simulink model "hp_v2"  (R2024b)
settings: Solver=VariableStepAuto  StartTime=0.0  StopTime=tf  MaxStep=1e-4  RelTol=1e-4  AbsTol=1e-4
values from neighbouring files (symbols this model uses):
  base = hexapod.base    [calcHomePose.m]    (also in calcMotorAngles.m; calcMotorAngles2.m; fk_z.m; ik_hexapod.m)
  coupler = hexapod.coupler    [calcHomePose.m]    (also in calcMotorAngles.m; calcMotorAngles2.m; fk_z.m; ik_hexapod.m)
  D = 2 * zeta * w_n * J_e    [simParams.m]
  excenter = hexapod.excenter    [calcHomePose.m]    (also in calcMotorAngles.m; calcMotorAngles2.m; fk_z.m; ik_hexapod.m)
  hexapod = get_params()    [A_LaiPresentation.m]    (also in Laga1D.m; bench_test.m; del_f.m; fk_z.m)
  m = platform_mass/6    [Laga1D.m]
  motorAngles = generateMotorData(pose, hexapod)    [A_LaiPresentation.m]    (also in Laga1D.m; calcMotorAngles.m = -(asin(g ./ (sqrt(ek.^2 + fk.^2)) ) - atan2(fk, ek)); calcMotorAngles2.m = (asin(g ./ (sqrt(ek.^2 + fk.^2)) ) - atan2(fk, ek)); fun_main.m)
  N = end_idx - start_idx + 1    [acc_solver.m]    (also in genaratePoseTK.m = length(data); ikd_lagrangian.m = size(q_traj, 1); simParams.m = 9)
  P = w_n^2 * J_e - K_e    [simParams.m]
  platform = hexapod.platform    [calcHomePose.m]    (also in calcMotorAngles.m; calcMotorAngles2.m; fk_z.m; ik_hexapod.m)
  platform_mass = 30    [simParams.m]
  radius = 0.01    [simParams.m]
  s = tf('s')    [S_curve.m]    (also in genPose.m = (-g + gm)/2 * t.^2 - gm * (p/2/pi)^2 * cos(2*pi/p*t+phi0) + )
  w_f = w_n * 10    (= 418.879020479)    [simParams.m]
  Z = fft(z)*2/length(z)    [modded_traj.m]
undefined symbols (not defined in the file or in its folder): X, Y
libraries: sm_lib x52, nesl_utility x41
(part 2 of 2)

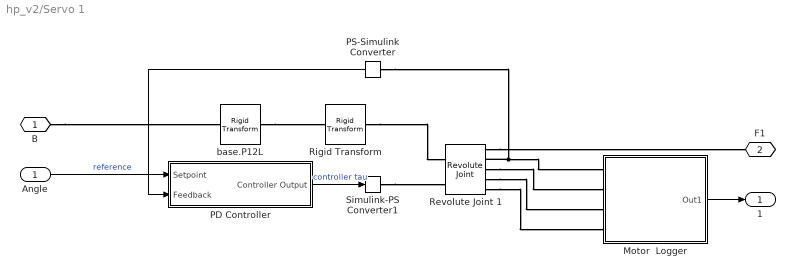
== system hp_v2/Servo 1 ==
  Angle : Inport
  Motor  Logger : Subsystem
  PD Controller : Subsystem
  PS-Simulink Converter : nesl_utility/PS-Simulink Converter  PhysicalDomain=network_engine_domain  SubClassName=ps_output  LeftPortType=input  RightPortType=output  PseudoPeriodic=off  Frequencies=[]  VectorFormat=inherit  Unit=inherit  AffineConversion=off
  Revolute Joint 1 : sm_lib/Joints/Revolute Joint  JointMode=Normal  CompositeWrenchDir=FollowerOnBase  CompositeWrenchFrame=BaseFrame  SenseConstraintForce=off  SenseConstraintTorque=off  SenseTotalForce=off  SenseTotalTorque=off  PositionTargetSpecify=on  PositionTargetPriority=High  PositionTargetValue=0  PositionTargetValueUnits=deg  VelocityTargetSpecify=off  VelocityTargetPriority=High  VelocityTargetValue=0  VelocityTargetValueUnits=deg/s  EquilibriumPosition=angular_spring_offset  EquilibriumPositionUnits=rad  SpringStiffness=angular_spring_constant  SpringStiffnessUnits=N*m/rad  DampingCoefficient=0  DampingCoefficientUnits=N*m*s/rad  LowerLimitSpecify=off  LowerLimitBound=-90  LowerLimitBoundUnits=deg  LowerLimitStiffness=1e4  LowerLimitStiffnessUnits=N*m/deg  LowerLimitDamping=10  LowerLimitDampingUnits=N*m/(deg/s)  LowerLimitTransitionRegionWidth=0.1  LowerLimitTransitionRegionWidthUnits=deg  UpperLimitSpecify=off  UpperLimitBound=90  UpperLimitBoundUnits=deg  UpperLimitStiffness=1e4  UpperLimitStiffnessUnits=N*m/deg  UpperLimitDamping=10  UpperLimitDampingUnits=N*m/(deg/s)  UpperLimitTransitionRegionWidth=0.1  UpperLimitTransitionRegionWidthUnits=deg  TorqueActuationMode=InputTorque  MotionActuationMode=ComputedMotion  SensePosition=on  SenseVelocity=on  SenseAcceleration=on  SenseTorqueForce=on  SenseLowerLimitTorqueForce=off  SenseUpperLimitTorqueForce=off
  Rigid Transform : sm_lib/Frames and Transforms/Rigid Transform  RotationMethod=StandardAxis  FollAlignAxisA=+X  BaseAlignAxisA=+Y  FollAlignAxisB=+Y  BaseAlignAxisB=+Z  RotationStandardAxis=+Z  RotationAngle=excenter.phi  RotationAngleUnits=rad  RotationArbitraryAxis=[0 0 1]  RotationSequenceAxes=FollowerAxes  RotationSequence=XYX  RotationSequenceAngles=[0 0 0]  RotationSequenceAnglesUnits=deg  RotationMatrix=[1 0 0;0 1 0;0 0 1]  Quaternion=[1 0 0 0]  TranslationMethod=None  TranslationCartesianOffset=[0 0 0]  TranslationCartesianOffsetUnits=m  TranslationStandardAxis=+Z  TranslationStandardOffset=0  TranslationStandardOffsetUnits=m  TranslationROffset=0  TranslationROffsetUnits=m  TranslationThetaOffset=0  TranslationThetaOffsetUnits=deg  TranslationZOffset=0  TranslationZOffsetUnits=m
  Simulink-PS Converter1 : nesl_utility/Simulink-PS Converter  PhysicalDomain=network_engine_domain  SubClassName=ps_input  LeftPortType=input  RightPortType=output  PseudoPeriodic=off  Frequencies=[]  NoiseDistribution=none  NoiseParameters=[]  Unit=1  AffineConversion=off  FilteringAndDerivatives=provide  SimscapeFilterOrder=1  InputFilterTimeConstant=0.001  UdotUserProvided=0
  base.P12L : sm_lib/Frames and Transforms/Rigid Transform  RotationMethod=StandardAxis  FollAlignAxisA=+X  BaseAlignAxisA=+Y  FollAlignAxisB=+Y  BaseAlignAxisB=+Z  RotationStandardAxis=+Y  RotationAngle=base.beta_sim(1)  RotationAngleUnits=rad  RotationArbitraryAxis=[0 0 1]  RotationSequenceAxes=FollowerAxes  RotationSequence=XYX  RotationSequenceAngles=[0 0 0]  RotationSequenceAnglesUnits=deg  RotationMatrix=[1 0 0;0 1 0;0 0 1]  Quaternion=[1 0 0 0]  TranslationMethod=Cartesian  TranslationCartesianOffset=base.P12L  TranslationCartesianOffsetUnits=m  TranslationStandardAxis=+Z  TranslationStandardOffset=0  TranslationStandardOffsetUnits=m  TranslationROffset=0  TranslationROffsetUnits=m  TranslationThetaOffset=0  TranslationThetaOffsetUnits=deg  TranslationZOffset=0  TranslationZOffsetUnits=m
  B : PMIOPort  Side=Left
  F1 : PMIOPort  Port=2  Side=Right
  1 : Outport
  wires:
  PS-Simulink Converter/1 -> PD Controller/2(Feedback)
  Angle/1 -> PD Controller/1(Setpoint)  "reference"
  PD Controller/1(Controller Output) -> Simulink-PS Converter1/1  "controller tau"
  Motor  Logger/1(Out1) -> 1/1
  connections:
  Revolute Joint 1/RConn1 -- F1/RConn1
  Revolute Joint 1/RConn5 -- Motor  Logger/LConn4
  PS-Simulink Converter/LConn1 -- Motor  Logger/LConn1 -- Revolute Joint 1/RConn2
  Simulink-PS Converter1/RConn1 -- Revolute Joint 1/LConn2
  base.P12L/RConn1 -- Rigid Transform/LConn1
  B/RConn1 -- base.P12L/LConn1
  Revolute Joint 1/RConn3 -- Motor  Logger/LConn2
  Revolute Joint 1/RConn4 -- Motor  Logger/LConn3
  Rigid Transform/RConn1 -- Revolute Joint 1/LConn1

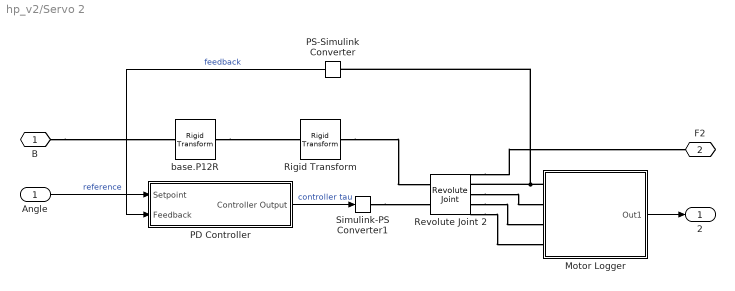
== system hp_v2/Servo 2 ==
  Angle : Inport
  Motor Logger : Subsystem
  PD Controller : Subsystem
  PS-Simulink Converter : nesl_utility/PS-Simulink Converter  PhysicalDomain=network_engine_domain  SubClassName=ps_output  LeftPortType=input  RightPortType=output  PseudoPeriodic=off  Frequencies=[]  VectorFormat=inherit  Unit=inherit  AffineConversion=off
  Revolute Joint 2 : sm_lib/Joints/Revolute Joint  JointMode=Normal  CompositeWrenchDir=FollowerOnBase  CompositeWrenchFrame=BaseFrame  SenseConstraintForce=off  SenseConstraintTorque=off  SenseTotalForce=off  SenseTotalTorque=off  PositionTargetSpecify=on  PositionTargetPriority=High  PositionTargetValue=0  PositionTargetValueUnits=deg  VelocityTargetSpecify=off  VelocityTargetPriority=High  VelocityTargetValue=0  VelocityTargetValueUnits=deg/s  EquilibriumPosition=angular_spring_offset  EquilibriumPositionUnits=rad  SpringStiffness=angular_spring_constant  SpringStiffnessUnits=N*m/rad  DampingCoefficient=0  DampingCoefficientUnits=N*m/(deg/s)  LowerLimitSpecify=off  LowerLimitBound=-90  LowerLimitBoundUnits=deg  LowerLimitStiffness=1e4  LowerLimitStiffnessUnits=N*m/deg  LowerLimitDamping=10  LowerLimitDampingUnits=N*m/(deg/s)  LowerLimitTransitionRegionWidth=0.1  LowerLimitTransitionRegionWidthUnits=deg  UpperLimitSpecify=off  UpperLimitBound=90  UpperLimitBoundUnits=deg  UpperLimitStiffness=1e4  UpperLimitStiffnessUnits=N*m/deg  UpperLimitDamping=10  UpperLimitDampingUnits=N*m/(deg/s)  UpperLimitTransitionRegionWidth=0.1  UpperLimitTransitionRegionWidthUnits=deg  TorqueActuationMode=InputTorque  MotionActuationMode=ComputedMotion  SensePosition=on  SenseVelocity=on  SenseAcceleration=on  SenseTorqueForce=on  SenseLowerLimitTorqueForce=off  SenseUpperLimitTorqueForce=off
  Rigid Transform : sm_lib/Frames and Transforms/Rigid Transform  RotationMethod=StandardAxis  FollAlignAxisA=+X  BaseAlignAxisA=+Y  FollAlignAxisB=+Y  BaseAlignAxisB=+Z  RotationStandardAxis=+Z  RotationAngle=excenter.phi  RotationAngleUnits=rad  RotationArbitraryAxis=[0 0 1]  RotationSequenceAxes=FollowerAxes  RotationSequence=XYX  RotationSequenceAngles=[0 0 0]  RotationSequenceAnglesUnits=deg  RotationMatrix=[1 0 0;0 1 0;0 0 1]  Quaternion=[1 0 0 0]  TranslationMethod=None  TranslationCartesianOffset=[0 0 0]  TranslationCartesianOffsetUnits=m  TranslationStandardAxis=+Z  TranslationStandardOffset=0  TranslationStandardOffsetUnits=m  TranslationROffset=0  TranslationROffsetUnits=m  TranslationThetaOffset=0  TranslationThetaOffsetUnits=deg  TranslationZOffset=0  TranslationZOffsetUnits=m
  Simulink-PS Converter1 : nesl_utility/Simulink-PS Converter  PhysicalDomain=network_engine_domain  SubClassName=ps_input  LeftPortType=input  RightPortType=output  PseudoPeriodic=off  Frequencies=[]  NoiseDistribution=none  NoiseParameters=[]  Unit=1  AffineConversion=off  FilteringAndDerivatives=provide  SimscapeFilterOrder=1  InputFilterTimeConstant=0.001  UdotUserProvided=0
  base.P12R : sm_lib/Frames and Transforms/Rigid Transform  RotationMethod=StandardAxis  FollAlignAxisA=+X  BaseAlignAxisA=+Y  FollAlignAxisB=+Y  BaseAlignAxisB=+Z  RotationStandardAxis=+Y  RotationAngle=base.beta_sim(2)  RotationAngleUnits=rad  RotationArbitraryAxis=[0 0 1]  RotationSequenceAxes=FollowerAxes  RotationSequence=XYX  RotationSequenceAngles=[0 0 0]  RotationSequenceAnglesUnits=deg  RotationMatrix=[1 0 0;0 1 0;0 0 1]  Quaternion=[1 0 0 0]  TranslationMethod=Cartesian  TranslationCartesianOffset=base.P12R  TranslationCartesianOffsetUnits=m  TranslationStandardAxis=+Z  TranslationStandardOffset=0  TranslationStandardOffsetUnits=m  TranslationROffset=0  TranslationROffsetUnits=m  TranslationThetaOffset=0  TranslationThetaOffsetUnits=deg  TranslationZOffset=0  TranslationZOffsetUnits=m
  B : PMIOPort  Side=Left
  F2 : PMIOPort  Port=2  Side=Right
  2 : Outport
  wires:
  Angle/1 -> PD Controller/1(Setpoint)  "reference"
  PD Controller/1(Controller Output) -> Simulink-PS Converter1/1  "controller tau"
  PS-Simulink Converter/1 -> PD Controller/2(Feedback)  "feedback"
  Motor Logger/1(Out1) -> 2/1
  connections:
  Revolute Joint 2/RConn1 -- F2/RConn1
  base.P12R/RConn1 -- Rigid Transform/LConn1
  Revolute Joint 2/RConn5 -- Motor Logger/LConn4
  Simulink-PS Converter1/RConn1 -- Revolute Joint 2/LConn2
  B/RConn1 -- base.P12R/LConn1
  Revolute Joint 2/RConn3 -- Motor Logger/LConn2
  Revolute Joint 2/RConn4 -- Motor Logger/LConn3
  Motor Logger/LConn1 -- PS-Simulink Converter/LConn1 -- Revolute Joint 2/RConn2
  Rigid Transform/RConn1 -- Revolute Joint 2/LConn1

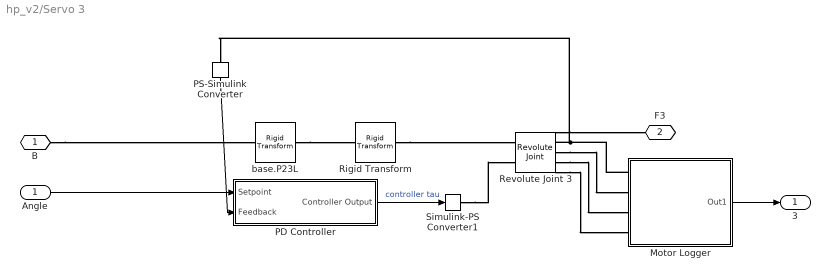
== system hp_v2/Servo 3 ==
  Angle : Inport
  Motor Logger : Subsystem
  PD Controller : Subsystem
  PS-Simulink Converter : nesl_utility/PS-Simulink Converter  PhysicalDomain=network_engine_domain  SubClassName=ps_output  LeftPortType=input  RightPortType=output  PseudoPeriodic=off  Frequencies=[]  VectorFormat=inherit  Unit=inherit  AffineConversion=off
  Revolute Joint 3 : sm_lib/Joints/Revolute Joint  JointMode=Normal  CompositeWrenchDir=FollowerOnBase  CompositeWrenchFrame=BaseFrame  SenseConstraintForce=off  SenseConstraintTorque=off  SenseTotalForce=off  SenseTotalTorque=off  PositionTargetSpecify=on  PositionTargetPriority=High  PositionTargetValue=0  PositionTargetValueUnits=deg  VelocityTargetSpecify=off  VelocityTargetPriority=High  VelocityTargetValue=0  VelocityTargetValueUnits=deg/s  EquilibriumPosition=angular_spring_offset  EquilibriumPositionUnits=rad  SpringStiffness=angular_spring_constant  SpringStiffnessUnits=N*m/rad  DampingCoefficient=0  DampingCoefficientUnits=N*m/(deg/s)  LowerLimitSpecify=off  LowerLimitBound=-90  LowerLimitBoundUnits=deg  LowerLimitStiffness=1e4  LowerLimitStiffnessUnits=N*m/deg  LowerLimitDamping=10  LowerLimitDampingUnits=N*m/(deg/s)  LowerLimitTransitionRegionWidth=0.1  LowerLimitTransitionRegionWidthUnits=deg  UpperLimitSpecify=off  UpperLimitBound=90  UpperLimitBoundUnits=deg  UpperLimitStiffness=1e4  UpperLimitStiffnessUnits=N*m/deg  UpperLimitDamping=10  UpperLimitDampingUnits=N*m/(deg/s)  UpperLimitTransitionRegionWidth=0.1  UpperLimitTransitionRegionWidthUnits=deg  TorqueActuationMode=InputTorque  MotionActuationMode=ComputedMotion  SensePosition=on  SenseVelocity=on  SenseAcceleration=on  SenseTorqueForce=on  SenseLowerLimitTorqueForce=off  SenseUpperLimitTorqueForce=off
  Rigid Transform : sm_lib/Frames and Transforms/Rigid Transform  RotationMethod=StandardAxis  FollAlignAxisA=+X  BaseAlignAxisA=+Y  FollAlignAxisB=+Y  BaseAlignAxisB=+Z  RotationStandardAxis=+Z  RotationAngle=excenter.phi  RotationAngleUnits=rad  RotationArbitraryAxis=[0 0 1]  RotationSequenceAxes=FollowerAxes  RotationSequence=XYX  RotationSequenceAngles=[0 0 0]  RotationSequenceAnglesUnits=deg  RotationMatrix=[1 0 0;0 1 0;0 0 1]  Quaternion=[1 0 0 0]  TranslationMethod=None  TranslationCartesianOffset=[0 0 0]  TranslationCartesianOffsetUnits=m  TranslationStandardAxis=+Z  TranslationStandardOffset=0  TranslationStandardOffsetUnits=m  TranslationROffset=0  TranslationROffsetUnits=m  TranslationThetaOffset=0  TranslationThetaOffsetUnits=deg  TranslationZOffset=0  TranslationZOffsetUnits=m
  Simulink-PS Converter1 : nesl_utility/Simulink-PS Converter  PhysicalDomain=network_engine_domain  SubClassName=ps_input  LeftPortType=input  RightPortType=output  PseudoPeriodic=off  Frequencies=[]  NoiseDistribution=none  NoiseParameters=[]  Unit=1  AffineConversion=off  FilteringAndDerivatives=provide  SimscapeFilterOrder=1  InputFilterTimeConstant=0.001  UdotUserProvided=0
  base.P23L : sm_lib/Frames and Transforms/Rigid Transform  RotationMethod=StandardAxis  FollAlignAxisA=+X  BaseAlignAxisA=+Y  FollAlignAxisB=+Y  BaseAlignAxisB=+Z  RotationStandardAxis=+Y  RotationAngle=base.beta_sim(3)  RotationAngleUnits=rad  RotationArbitraryAxis=[0 0 1]  RotationSequenceAxes=FollowerAxes  RotationSequence=XYX  RotationSequenceAngles=[0 0 0]  RotationSequenceAnglesUnits=deg  RotationMatrix=[1 0 0;0 1 0;0 0 1]  Quaternion=[1 0 0 0]  TranslationMethod=Cartesian  TranslationCartesianOffset=base.P23L  TranslationCartesianOffsetUnits=m  TranslationStandardAxis=+Z  TranslationStandardOffset=0  TranslationStandardOffsetUnits=m  TranslationROffset=0  TranslationROffsetUnits=m  TranslationThetaOffset=0  TranslationThetaOffsetUnits=deg  TranslationZOffset=0  TranslationZOffsetUnits=m
  B : PMIOPort  Side=Left
  F3 : PMIOPort  Port=2  Side=Right
  3 : Outport
  wires:
  Motor Logger/1(Out1) -> 3/1
  Angle/1 -> PD Controller/1(Setpoint)
  PS-Simulink Converter/1 -> PD Controller/2(Feedback)
  PD Controller/1(Controller Output) -> Simulink-PS Converter1/1  "controller tau"
  connections:
  Revolute Joint 3/RConn5 -- Motor Logger/LConn4
  Revolute Joint 3/RConn4 -- Motor Logger/LConn3
  Simulink-PS Converter1/RConn1 -- Revolute Joint 3/LConn2
  Revolute Joint 3/RConn3 -- Motor Logger/LConn2
  B/RConn1 -- base.P23L/LConn1
  Revolute Joint 3/RConn1 -- F3/RConn1
  Rigid Transform/RConn1 -- Revolute Joint 3/LConn1
  Motor Logger/LConn1 -- PS-Simulink Converter/LConn1 -- Revolute Joint 3/RConn2
  base.P23L/RConn1 -- Rigid Transform/LConn1

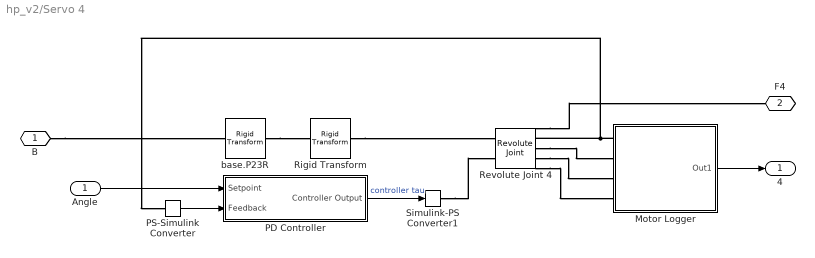
== system hp_v2/Servo 4 ==
  Angle : Inport
  Motor Logger : Subsystem
  PD Controller : Subsystem
  PS-Simulink Converter : nesl_utility/PS-Simulink Converter  PhysicalDomain=network_engine_domain  SubClassName=ps_output  LeftPortType=input  RightPortType=output  PseudoPeriodic=off  Frequencies=[]  VectorFormat=inherit  Unit=inherit  AffineConversion=off
  Revolute Joint 4 : sm_lib/Joints/Revolute Joint  JointMode=Normal  CompositeWrenchDir=FollowerOnBase  CompositeWrenchFrame=BaseFrame  SenseConstraintForce=off  SenseConstraintTorque=off  SenseTotalForce=off  SenseTotalTorque=off  PositionTargetSpecify=on  PositionTargetPriority=High  PositionTargetValue=0  PositionTargetValueUnits=deg  VelocityTargetSpecify=off  VelocityTargetPriority=High  VelocityTargetValue=0  VelocityTargetValueUnits=deg/s  EquilibriumPosition=angular_spring_offset  EquilibriumPositionUnits=rad  SpringStiffness=angular_spring_constant  SpringStiffnessUnits=N*m/rad  DampingCoefficient=0  DampingCoefficientUnits=N*m/(deg/s)  LowerLimitSpecify=off  LowerLimitBound=-90  LowerLimitBoundUnits=deg  LowerLimitStiffness=1e4  LowerLimitStiffnessUnits=N*m/deg  LowerLimitDamping=10  LowerLimitDampingUnits=N*m/(deg/s)  LowerLimitTransitionRegionWidth=0.1  LowerLimitTransitionRegionWidthUnits=deg  UpperLimitSpecify=off  UpperLimitBound=90  UpperLimitBoundUnits=deg  UpperLimitStiffness=1e4  UpperLimitStiffnessUnits=N*m/deg  UpperLimitDamping=10  UpperLimitDampingUnits=N*m/(deg/s)  UpperLimitTransitionRegionWidth=0.1  UpperLimitTransitionRegionWidthUnits=deg  TorqueActuationMode=InputTorque  MotionActuationMode=ComputedMotion  SensePosition=on  SenseVelocity=on  SenseAcceleration=on  SenseTorqueForce=on  SenseLowerLimitTorqueForce=off  SenseUpperLimitTorqueForce=off
  Rigid Transform : sm_lib/Frames and Transforms/Rigid Transform  RotationMethod=StandardAxis  FollAlignAxisA=+X  BaseAlignAxisA=+Y  FollAlignAxisB=+Y  BaseAlignAxisB=+Z  RotationStandardAxis=+Z  RotationAngle=excenter.phi  RotationAngleUnits=rad  RotationArbitraryAxis=[0 0 1]  RotationSequenceAxes=FollowerAxes  RotationSequence=XYX  RotationSequenceAngles=[0 0 0]  RotationSequenceAnglesUnits=deg  RotationMatrix=[1 0 0;0 1 0;0 0 1]  Quaternion=[1 0 0 0]  TranslationMethod=None  TranslationCartesianOffset=[0 0 0]  TranslationCartesianOffsetUnits=m  TranslationStandardAxis=+Z  TranslationStandardOffset=0  TranslationStandardOffsetUnits=m  TranslationROffset=0  TranslationROffsetUnits=m  TranslationThetaOffset=0  TranslationThetaOffsetUnits=deg  TranslationZOffset=0  TranslationZOffsetUnits=m
  Simulink-PS Converter1 : nesl_utility/Simulink-PS Converter  PhysicalDomain=network_engine_domain  SubClassName=ps_input  LeftPortType=input  RightPortType=output  PseudoPeriodic=off  Frequencies=[]  NoiseDistribution=none  NoiseParameters=[]  Unit=1  AffineConversion=off  FilteringAndDerivatives=provide  SimscapeFilterOrder=1  InputFilterTimeConstant=0.001  UdotUserProvided=0
  base.P23R : sm_lib/Frames and Transforms/Rigid Transform  RotationMethod=StandardAxis  FollAlignAxisA=+X  BaseAlignAxisA=+Y  FollAlignAxisB=+Y  BaseAlignAxisB=+Z  RotationStandardAxis=+Y  RotationAngle=base.beta_sim(4)  RotationAngleUnits=rad  RotationArbitraryAxis=[0 0 1]  RotationSequenceAxes=FollowerAxes  RotationSequence=XYX  RotationSequenceAngles=[0 0 0]  RotationSequenceAnglesUnits=deg  RotationMatrix=[1 0 0;0 1 0;0 0 1]  Quaternion=[1 0 0 0]  TranslationMethod=Cartesian  TranslationCartesianOffset=base.P23R  TranslationCartesianOffsetUnits=m  TranslationStandardAxis=+Z  TranslationStandardOffset=0  TranslationStandardOffsetUnits=m  TranslationROffset=0  TranslationROffsetUnits=m  TranslationThetaOffset=0  TranslationThetaOffsetUnits=deg  TranslationZOffset=0  TranslationZOffsetUnits=m
  B : PMIOPort  Side=Left
  F4 : PMIOPort  Port=2  Side=Right
  4 : Outport
  wires:
  PD Controller/1(Controller Output) -> Simulink-PS Converter1/1  "controller tau"
  Motor Logger/1(Out1) -> 4/1
  Angle/1 -> PD Controller/1(Setpoint)
  PS-Simulink Converter/1 -> PD Controller/2(Feedback)
  connections:
  Revolute Joint 4/RConn4 -- Motor Logger/LConn3
  B/RConn1 -- base.P23R/LConn1
  base.P23R/RConn1 -- Rigid Transform/LConn1
  Revolute Joint 4/RConn3 -- Motor Logger/LConn2
  Simulink-PS Converter1/RConn1 -- Revolute Joint 4/LConn2
  Revolute Joint 4/RConn5 -- Motor Logger/LConn4
  Revolute Joint 4/RConn1 -- F4/RConn1
  Motor Logger/LConn1 -- PS-Simulink Converter/LConn1 -- Revolute Joint 4/RConn2
  Rigid Transform/RConn1 -- Revolute Joint 4/LConn1

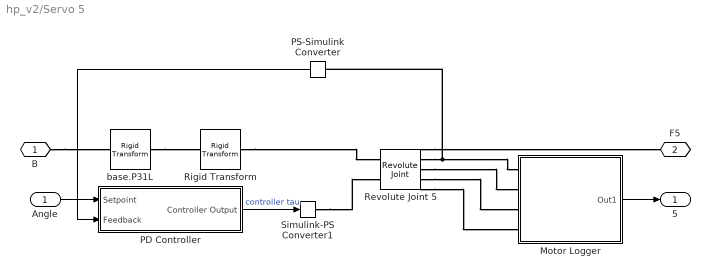
== system hp_v2/Servo 5 ==
  Angle : Inport
  Motor Logger : Subsystem
  PD Controller : Subsystem
  PS-Simulink Converter : nesl_utility/PS-Simulink Converter  PhysicalDomain=network_engine_domain  SubClassName=ps_output  LeftPortType=input  RightPortType=output  PseudoPeriodic=off  Frequencies=[]  VectorFormat=inherit  Unit=inherit  AffineConversion=off
  Revolute Joint 5 : sm_lib/Joints/Revolute Joint  JointMode=Normal  CompositeWrenchDir=FollowerOnBase  CompositeWrenchFrame=BaseFrame  SenseConstraintForce=off  SenseConstraintTorque=off  SenseTotalForce=off  SenseTotalTorque=off  PositionTargetSpecify=on  PositionTargetPriority=High  PositionTargetValue=0  PositionTargetValueUnits=deg  VelocityTargetSpecify=off  VelocityTargetPriority=High  VelocityTargetValue=0  VelocityTargetValueUnits=deg/s  EquilibriumPosition=angular_spring_offset  EquilibriumPositionUnits=rad  SpringStiffness=angular_spring_constant  SpringStiffnessUnits=N*m/rad  DampingCoefficient=0  DampingCoefficientUnits=N*m/(deg/s)  LowerLimitSpecify=off  LowerLimitBound=-90  LowerLimitBoundUnits=deg  LowerLimitStiffness=1e4  LowerLimitStiffnessUnits=N*m/deg  LowerLimitDamping=10  LowerLimitDampingUnits=N*m/(deg/s)  LowerLimitTransitionRegionWidth=0.1  LowerLimitTransitionRegionWidthUnits=deg  UpperLimitSpecify=off  UpperLimitBound=90  UpperLimitBoundUnits=deg  UpperLimitStiffness=1e4  UpperLimitStiffnessUnits=N*m/deg  UpperLimitDamping=10  UpperLimitDampingUnits=N*m/(deg/s)  UpperLimitTransitionRegionWidth=0.1  UpperLimitTransitionRegionWidthUnits=deg  TorqueActuationMode=InputTorque  MotionActuationMode=ComputedMotion  SensePosition=on  SenseVelocity=on  SenseAcceleration=on  SenseTorqueForce=on  SenseLowerLimitTorqueForce=off  SenseUpperLimitTorqueForce=off
  Rigid Transform : sm_lib/Frames and Transforms/Rigid Transform  RotationMethod=StandardAxis  FollAlignAxisA=+X  BaseAlignAxisA=+Y  FollAlignAxisB=+Y  BaseAlignAxisB=+Z  RotationStandardAxis=+Z  RotationAngle=excenter.phi  RotationAngleUnits=rad  RotationArbitraryAxis=[0 0 1]  RotationSequenceAxes=FollowerAxes  RotationSequence=XYX  RotationSequenceAngles=[0 0 0]  RotationSequenceAnglesUnits=deg  RotationMatrix=[1 0 0;0 1 0;0 0 1]  Quaternion=[1 0 0 0]  TranslationMethod=None  TranslationCartesianOffset=[0 0 0]  TranslationCartesianOffsetUnits=m  TranslationStandardAxis=+Z  TranslationStandardOffset=0  TranslationStandardOffsetUnits=m  TranslationROffset=0  TranslationROffsetUnits=m  TranslationThetaOffset=0  TranslationThetaOffsetUnits=deg  TranslationZOffset=0  TranslationZOffsetUnits=m
  Simulink-PS Converter1 : nesl_utility/Simulink-PS Converter  PhysicalDomain=network_engine_domain  SubClassName=ps_input  LeftPortType=input  RightPortType=output  PseudoPeriodic=off  Frequencies=[]  NoiseDistribution=none  NoiseParameters=[]  Unit=1  AffineConversion=off  FilteringAndDerivatives=provide  SimscapeFilterOrder=1  InputFilterTimeConstant=0.001  UdotUserProvided=0
  base.P31L : sm_lib/Frames and Transforms/Rigid Transform  RotationMethod=StandardAxis  FollAlignAxisA=+X  BaseAlignAxisA=+Y  FollAlignAxisB=+Y  BaseAlignAxisB=+Z  RotationStandardAxis=+Y  RotationAngle=base.beta_sim(5)  RotationAngleUnits=rad  RotationArbitraryAxis=[0 0 1]  RotationSequenceAxes=FollowerAxes  RotationSequence=XYX  RotationSequenceAngles=[0 0 0]  RotationSequenceAnglesUnits=deg  RotationMatrix=[1 0 0;0 1 0;0 0 1]  Quaternion=[1 0 0 0]  TranslationMethod=Cartesian  TranslationCartesianOffset=base.P31L  TranslationCartesianOffsetUnits=m  TranslationStandardAxis=+Z  TranslationStandardOffset=0  TranslationStandardOffsetUnits=m  TranslationROffset=0  TranslationROffsetUnits=m  TranslationThetaOffset=0  TranslationThetaOffsetUnits=deg  TranslationZOffset=0  TranslationZOffsetUnits=m
  B : PMIOPort  Side=Left
  F5 : PMIOPort  Port=2  Side=Right
  5 : Outport
  wires:
  Angle/1 -> PD Controller/1(Setpoint)
  PD Controller/1(Controller Output) -> Simulink-PS Converter1/1  "controller tau"
  PS-Simulink Converter/1 -> PD Controller/2(Feedback)
  Motor Logger/1(Out1) -> 5/1
  connections:
  B/RConn1 -- base.P31L/LConn1
  Revolute Joint 5/RConn2 -- Motor Logger/LConn1 -- PS-Simulink Converter/LConn1
  base.P31L/RConn1 -- Rigid Transform/LConn1
  Simulink-PS Converter1/RConn1 -- Revolute Joint 5/LConn2
  Revolute Joint 5/RConn1 -- F5/RConn1
  Revolute Joint 5/RConn3 -- Motor Logger/LConn2
  Revolute Joint 5/RConn4 -- Motor Logger/LConn3
  Revolute Joint 5/RConn5 -- Motor Logger/LConn4
  Rigid Transform/RConn1 -- Revolute Joint 5/LConn1

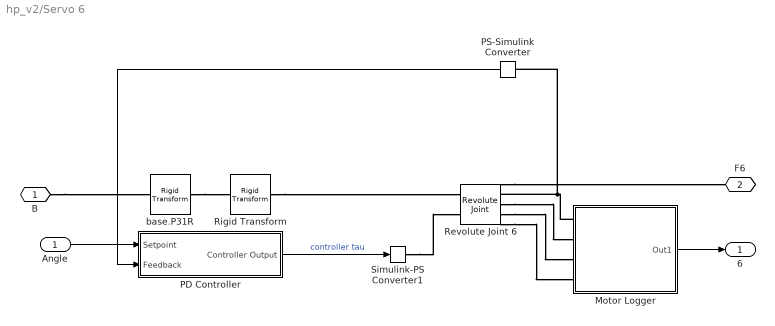
== system hp_v2/Servo 6 ==
  Angle : Inport
  Motor Logger : Subsystem
  PD Controller : Subsystem
  PS-Simulink Converter : nesl_utility/PS-Simulink Converter  PhysicalDomain=network_engine_domain  SubClassName=ps_output  LeftPortType=input  RightPortType=output  PseudoPeriodic=off  Frequencies=[]  VectorFormat=inherit  Unit=inherit  AffineConversion=off
  Revolute Joint 6 : sm_lib/Joints/Revolute Joint  JointMode=Normal  CompositeWrenchDir=FollowerOnBase  CompositeWrenchFrame=BaseFrame  SenseConstraintForce=off  SenseConstraintTorque=off  SenseTotalForce=off  SenseTotalTorque=off  PositionTargetSpecify=on  PositionTargetPriority=High  PositionTargetValue=0  PositionTargetValueUnits=deg  VelocityTargetSpecify=off  VelocityTargetPriority=High  VelocityTargetValue=0  VelocityTargetValueUnits=deg/s  EquilibriumPosition=angular_spring_offset  EquilibriumPositionUnits=rad  SpringStiffness=angular_spring_constant  SpringStiffnessUnits=N*m/rad  DampingCoefficient=0  DampingCoefficientUnits=N*m/(deg/s)  LowerLimitSpecify=off  LowerLimitBound=-90  LowerLimitBoundUnits=deg  LowerLimitStiffness=1e4  LowerLimitStiffnessUnits=N*m/deg  LowerLimitDamping=10  LowerLimitDampingUnits=N*m/(deg/s)  LowerLimitTransitionRegionWidth=0.1  LowerLimitTransitionRegionWidthUnits=deg  UpperLimitSpecify=off  UpperLimitBound=90  UpperLimitBoundUnits=deg  UpperLimitStiffness=1e4  UpperLimitStiffnessUnits=N*m/deg  UpperLimitDamping=10  UpperLimitDampingUnits=N*m/(deg/s)  UpperLimitTransitionRegionWidth=0.1  UpperLimitTransitionRegionWidthUnits=deg  TorqueActuationMode=InputTorque  MotionActuationMode=ComputedMotion  SensePosition=on  SenseVelocity=on  SenseAcceleration=on  SenseTorqueForce=on  SenseLowerLimitTorqueForce=off  SenseUpperLimitTorqueForce=off
  Rigid Transform : sm_lib/Frames and Transforms/Rigid Transform  RotationMethod=StandardAxis  FollAlignAxisA=+X  BaseAlignAxisA=+Y  FollAlignAxisB=+Y  BaseAlignAxisB=+Z  RotationStandardAxis=+Z  RotationAngle=excenter.phi  RotationAngleUnits=rad  RotationArbitraryAxis=[0 0 1]  RotationSequenceAxes=FollowerAxes  RotationSequence=XYX  RotationSequenceAngles=[0 0 0]  RotationSequenceAnglesUnits=deg  RotationMatrix=[1 0 0;0 1 0;0 0 1]  Quaternion=[1 0 0 0]  TranslationMethod=None  TranslationCartesianOffset=[0 0 0]  TranslationCartesianOffsetUnits=m  TranslationStandardAxis=+Z  TranslationStandardOffset=0  TranslationStandardOffsetUnits=m  TranslationROffset=0  TranslationROffsetUnits=m  TranslationThetaOffset=0  TranslationThetaOffsetUnits=deg  TranslationZOffset=0  TranslationZOffsetUnits=m
  Simulink-PS Converter1 : nesl_utility/Simulink-PS Converter  PhysicalDomain=network_engine_domain  SubClassName=ps_input  LeftPortType=input  RightPortType=output  PseudoPeriodic=off  Frequencies=[]  NoiseDistribution=none  NoiseParameters=[]  Unit=1  AffineConversion=off  FilteringAndDerivatives=provide  SimscapeFilterOrder=1  InputFilterTimeConstant=0.001  UdotUserProvided=0
  base.P31R : sm_lib/Frames and Transforms/Rigid Transform  RotationMethod=StandardAxis  FollAlignAxisA=+X  BaseAlignAxisA=+Y  FollAlignAxisB=+Y  BaseAlignAxisB=+Z  RotationStandardAxis=+Y  RotationAngle=base.beta_sim(6)  RotationAngleUnits=rad  RotationArbitraryAxis=[0 0 1]  RotationSequenceAxes=FollowerAxes  RotationSequence=XYX  RotationSequenceAngles=[0 0 0]  RotationSequenceAnglesUnits=deg  RotationMatrix=[1 0 0;0 1 0;0 0 1]  Quaternion=[1 0 0 0]  TranslationMethod=Cartesian  TranslationCartesianOffset=base.P31R  TranslationCartesianOffsetUnits=m  TranslationStandardAxis=+Z  TranslationStandardOffset=0  TranslationStandardOffsetUnits=m  TranslationROffset=0  TranslationROffsetUnits=m  TranslationThetaOffset=0  TranslationThetaOffsetUnits=deg  TranslationZOffset=0  TranslationZOffsetUnits=m
  B : PMIOPort  Side=Left
  F6 : PMIOPort  Port=2  Side=Right
  6 : Outport
  wires:
  PD Controller/1(Controller Output) -> Simulink-PS Converter1/1  "controller tau"
  Motor Logger/1(Out1) -> 6/1
  Angle/1 -> PD Controller/1(Setpoint)
  PS-Simulink Converter/1 -> PD Controller/2(Feedback)
  connections:
  Revolute Joint 6/RConn4 -- Motor Logger/LConn3
  B/RConn1 -- base.P31R/LConn1
  Motor Logger/LConn1 -- Revolute Joint 6/RConn2 -- PS-Simulink Converter/LConn1
  Revolute Joint 6/RConn5 -- Motor Logger/LConn4
  Revolute Joint 6/RConn1 -- F6/RConn1
  Rigid Transform/RConn1 -- Revolute Joint 6/LConn1
  Revolute Joint 6/RConn3 -- Motor Logger/LConn2
  Simulink-PS Converter1/RConn1 -- Revolute Joint 6/LConn2
  base.P31R/RConn1 -- Rigid Transform/LConn1

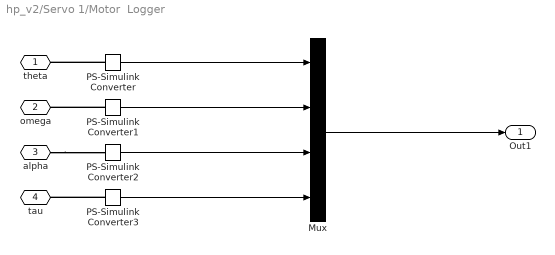
== system hp_v2/Servo 1/Motor  Logger ==
  Mux : Mux
  PS-Simulink Converter{,1..3} (4 alike) : nesl_utility/PS-Simulink Converter  PhysicalDomain=network_engine_domain  SubClassName=ps_output  LeftPortType=input  RightPortType=output  PseudoPeriodic=off  Frequencies=[]  VectorFormat=inherit  Unit=inherit  AffineConversion=off
  theta : PMIOPort  Side=Left
  omega : PMIOPort  Port=2  Side=Left
  alpha : PMIOPort  Port=3  Side=Left
  tau : PMIOPort  Port=4  Side=Left
  Out1 : Outport
  wires:
  PS-Simulink Converter/1 -> Mux/1
  PS-Simulink Converter1/1 -> Mux/2
  PS-Simulink Converter2/1 -> Mux/3
  PS-Simulink Converter3/1 -> Mux/4
  Mux/1 -> Out1/1
  connections:
  PS-Simulink Converter/LConn1 -- theta/RConn1
  PS-Simulink Converter1/LConn1 -- omega/RConn1
  alpha/RConn1 -- PS-Simulink Converter2/LConn1
  PS-Simulink Converter3/LConn1 -- tau/RConn1

== system hp_v2/Servo 1/PD Controller ==
  Setpoint : Inport
  Feedback : Inport  Port=2
  Differentiator : TransferFcn  Numerator=[D*w_f 0]  Denominator=[1 w_f]
  Gain : Gain  Gain=P
  Sum : Sum  Inputs=|+-
  Sum1 : Sum  Inputs=|++
  Controller Output : Outport
  wires:
  Differentiator/1 -> Sum1/2
  Setpoint/1 -> Sum/1
  Gain/1 -> Sum1/1
  Sum1/1 -> Controller Output/1
  Feedback/1 -> Sum/2
  Sum/1 -> Differentiator/1, Gain/1

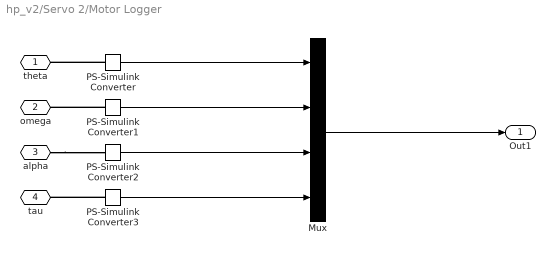
== system hp_v2/Servo 2/Motor Logger ==
  Mux : Mux
  PS-Simulink Converter{,1..3} (4 alike) : nesl_utility/PS-Simulink Converter  PhysicalDomain=network_engine_domain  SubClassName=ps_output  LeftPortType=input  RightPortType=output  PseudoPeriodic=off  Frequencies=[]  VectorFormat=inherit  Unit=inherit  AffineConversion=off
  theta : PMIOPort  Side=Left
  omega : PMIOPort  Port=2  Side=Left
  alpha : PMIOPort  Port=3  Side=Left
  tau : PMIOPort  Port=4  Side=Left
  Out1 : Outport
  wires:
  PS-Simulink Converter/1 -> Mux/1
  PS-Simulink Converter1/1 -> Mux/2
  PS-Simulink Converter2/1 -> Mux/3
  PS-Simulink Converter3/1 -> Mux/4
  Mux/1 -> Out1/1
  connections:
  PS-Simulink Converter/LConn1 -- theta/RConn1
  PS-Simulink Converter1/LConn1 -- omega/RConn1
  alpha/RConn1 -- PS-Simulink Converter2/LConn1
  PS-Simulink Converter3/LConn1 -- tau/RConn1

== system hp_v2/Servo 2/PD Controller ==
  Setpoint : Inport
  Feedback : Inport  Port=2
  Differentiator : TransferFcn  Numerator=[D*w_f 0]  Denominator=[1 w_f]
  Gain : Gain  Gain=P
  Sum : Sum  Inputs=|+-
  Sum1 : Sum  Inputs=|++
  Controller Output : Outport
  wires:
  Differentiator/1 -> Sum1/2
  Setpoint/1 -> Sum/1
  Gain/1 -> Sum1/1
  Sum1/1 -> Controller Output/1
  Feedback/1 -> Sum/2
  Sum/1 -> Differentiator/1, Gain/1

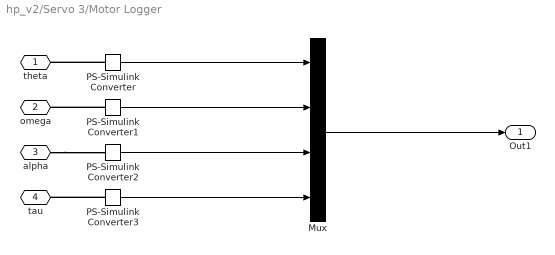
== system hp_v2/Servo 3/Motor Logger ==
  Mux : Mux
  PS-Simulink Converter{,1..3} (4 alike) : nesl_utility/PS-Simulink Converter  PhysicalDomain=network_engine_domain  SubClassName=ps_output  LeftPortType=input  RightPortType=output  PseudoPeriodic=off  Frequencies=[]  VectorFormat=inherit  Unit=inherit  AffineConversion=off
  theta : PMIOPort  Side=Left
  omega : PMIOPort  Port=2  Side=Left
  alpha : PMIOPort  Port=3  Side=Left
  tau : PMIOPort  Port=4  Side=Left
  Out1 : Outport
  wires:
  PS-Simulink Converter/1 -> Mux/1
  PS-Simulink Converter1/1 -> Mux/2
  PS-Simulink Converter2/1 -> Mux/3
  PS-Simulink Converter3/1 -> Mux/4
  Mux/1 -> Out1/1
  connections:
  PS-Simulink Converter/LConn1 -- theta/RConn1
  PS-Simulink Converter1/LConn1 -- omega/RConn1
  alpha/RConn1 -- PS-Simulink Converter2/LConn1
  PS-Simulink Converter3/LConn1 -- tau/RConn1

== system hp_v2/Servo 3/PD Controller ==
  Setpoint : Inport
  Feedback : Inport  Port=2
  Differentiator : TransferFcn  Numerator=[D*w_f 0]  Denominator=[1 w_f]
  Gain : Gain  Gain=P
  Sum : Sum  Inputs=|+-
  Sum1 : Sum  Inputs=|++
  Controller Output : Outport
  wires:
  Differentiator/1 -> Sum1/2
  Setpoint/1 -> Sum/1
  Gain/1 -> Sum1/1
  Sum1/1 -> Controller Output/1
  Feedback/1 -> Sum/2
  Sum/1 -> Differentiator/1, Gain/1

== system hp_v2/Servo 4/Motor Logger ==
  Mux : Mux
  PS-Simulink Converter{,1..3} (4 alike) : nesl_utility/PS-Simulink Converter  PhysicalDomain=network_engine_domain  SubClassName=ps_output  LeftPortType=input  RightPortType=output  PseudoPeriodic=off  Frequencies=[]  VectorFormat=inherit  Unit=inherit  AffineConversion=off
  theta : PMIOPort  Side=Left
  omega : PMIOPort  Port=2  Side=Left
  alpha : PMIOPort  Port=3  Side=Left
  tau : PMIOPort  Port=4  Side=Left
  Out1 : Outport
  wires:
  PS-Simulink Converter/1 -> Mux/1
  PS-Simulink Converter1/1 -> Mux/2
  PS-Simulink Converter2/1 -> Mux/3
  PS-Simulink Converter3/1 -> Mux/4
  Mux/1 -> Out1/1
  connections:
  PS-Simulink Converter/LConn1 -- theta/RConn1
  PS-Simulink Converter1/LConn1 -- omega/RConn1
  alpha/RConn1 -- PS-Simulink Converter2/LConn1
  PS-Simulink Converter3/LConn1 -- tau/RConn1

== system hp_v2/Servo 4/PD Controller ==
  Setpoint : Inport
  Feedback : Inport  Port=2
  Differentiator : TransferFcn  Numerator=[D*w_f 0]  Denominator=[1 w_f]
  Gain : Gain  Gain=P
  Sum : Sum  Inputs=|+-
  Sum1 : Sum  Inputs=|++
  Controller Output : Outport
  wires:
  Differentiator/1 -> Sum1/2
  Setpoint/1 -> Sum/1
  Gain/1 -> Sum1/1
  Sum1/1 -> Controller Output/1
  Feedback/1 -> Sum/2
  Sum/1 -> Differentiator/1, Gain/1

== system hp_v2/Servo 5/Motor Logger ==
  Mux : Mux
  PS-Simulink Converter{,1..3} (4 alike) : nesl_utility/PS-Simulink Converter  PhysicalDomain=network_engine_domain  SubClassName=ps_output  LeftPortType=input  RightPortType=output  PseudoPeriodic=off  Frequencies=[]  VectorFormat=inherit  Unit=inherit  AffineConversion=off
  theta : PMIOPort  Side=Left
  omega : PMIOPort  Port=2  Side=Left
  alpha : PMIOPort  Port=3  Side=Left
  tau : PMIOPort  Port=4  Side=Left
  Out1 : Outport
  wires:
  PS-Simulink Converter/1 -> Mux/1
  PS-Simulink Converter1/1 -> Mux/2
  PS-Simulink Converter2/1 -> Mux/3
  PS-Simulink Converter3/1 -> Mux/4
  Mux/1 -> Out1/1
  connections:
  PS-Simulink Converter/LConn1 -- theta/RConn1
  PS-Simulink Converter1/LConn1 -- omega/RConn1
  alpha/RConn1 -- PS-Simulink Converter2/LConn1
  PS-Simulink Converter3/LConn1 -- tau/RConn1

== system hp_v2/Servo 5/PD Controller ==
  Setpoint : Inport
  Feedback : Inport  Port=2
  Differentiator : TransferFcn  Numerator=[D*w_f 0]  Denominator=[1 w_f]
  Gain : Gain  Gain=P
  Sum : Sum  Inputs=|+-
  Sum1 : Sum  Inputs=|++
  Controller Output : Outport
  wires:
  Differentiator/1 -> Sum1/2
  Setpoint/1 -> Sum/1
  Gain/1 -> Sum1/1
  Sum1/1 -> Controller Output/1
  Feedback/1 -> Sum/2
  Sum/1 -> Differentiator/1, Gain/1

== system hp_v2/Servo 6/Motor Logger ==
  Mux : Mux
  PS-Simulink Converter{,1..3} (4 alike) : nesl_utility/PS-Simulink Converter  PhysicalDomain=network_engine_domain  SubClassName=ps_output  LeftPortType=input  RightPortType=output  PseudoPeriodic=off  Frequencies=[]  VectorFormat=inherit  Unit=inherit  AffineConversion=off
  theta : PMIOPort  Side=Left
  omega : PMIOPort  Port=2  Side=Left
  alpha : PMIOPort  Port=3  Side=Left
  tau : PMIOPort  Port=4  Side=Left
  Out1 : Outport
  wires:
  PS-Simulink Converter/1 -> Mux/1
  PS-Simulink Converter1/1 -> Mux/2
  PS-Simulink Converter2/1 -> Mux/3
  PS-Simulink Converter3/1 -> Mux/4
  Mux/1 -> Out1/1
  connections:
  PS-Simulink Converter/LConn1 -- theta/RConn1
  PS-Simulink Converter1/LConn1 -- omega/RConn1
  alpha/RConn1 -- PS-Simulink Converter2/LConn1
  PS-Simulink Converter3/LConn1 -- tau/RConn1

== system hp_v2/Servo 6/PD Controller ==
  Setpoint : Inport
  Feedback : Inport  Port=2
  Differentiator : TransferFcn  Numerator=[D*w_f 0]  Denominator=[1 w_f]
  Gain : Gain  Gain=P
  Sum : Sum  Inputs=|+-
  Sum1 : Sum  Inputs=|++
  Controller Output : Outport
  wires:
  Differentiator/1 -> Sum1/2
  Setpoint/1 -> Sum/1
  Gain/1 -> Sum1/1
  Sum1/1 -> Controller Output/1
  Feedback/1 -> Sum/2
  Sum/1 -> Differentiator/1, Gain/1

== matlab function hp_v2/MATLAB Function ==
  settings: updateMethod=DISCRETE  sampleTime=ts
  data: u input; tf input
function fcn(u, tf)
% Set the resolution for the progress bar
resolution = 5;  % Update progress bar every 5%

% Calculate the percentage complete
percentage = (u / tf) * 100;

% Check if the percentage is a multiple of the resolution
if mod(percentage, resolution) == 0
    % Calculate the number of dots based on the percentage
    strLength = 30;  % Total length of the progress bar
    nDots = floor(percentage / 100 * strLength);
    dotOut = ['[' repmat('=', 1, nDots) repmat('.', 1, strLength - nDots) ']'];
    percentageOut = sprintf(' : %3d%%', int32(floor(percentage)));

    % Create the output string with ">>" prefix
    strOut = ['>> ' dotOut percentageOut];

    % Print the progress bar
    fprintf('%s\n', strOut);  % Print each progress update on a new line
end

% Handle completion
if percentage >= 100
    fprintf('>> Simulation Complete.\n');
end
end
